simulink model "pv_partial_shading_control"  (R2021a)
settings: Solver=VariableStepAuto  StartTime=0.0  StopTime=2  RelTol=1e-3
libraries: pid_lib x5, spsSeriesRLCBranchLib x5, spsDiodeLib x4, spsabctodq0Lib x4, spsPVArrayLib x3, spsCurrentMeasurementLib x2, spsThreePhaseVIMeasurementLib x2, spsVoltageMeasurementLib x2, spsGroundLib x1, spsIGBTDiodeLib x1, spsPWMGenerator2LevelLib x1, spsPWMGeneratorDCDCLib x1
settings Model: Creator=30698  LastModifiedBy=30698
settings SolverCC: ZeroCrossAlgorithm=Adaptive
settings DebuggingCC: IgnoredZcDiagnostic=none  UnconnectedInputMsg=none  UnconnectedOutputMsg=none  UnconnectedLineMsg=none
settings ModelReferenceCC: EnableRefExpFcnMdlSchedulingChecks=off
settings RTWCC: Description=Generic Real-Time Target  DLArmComputeVersion=20.02.1

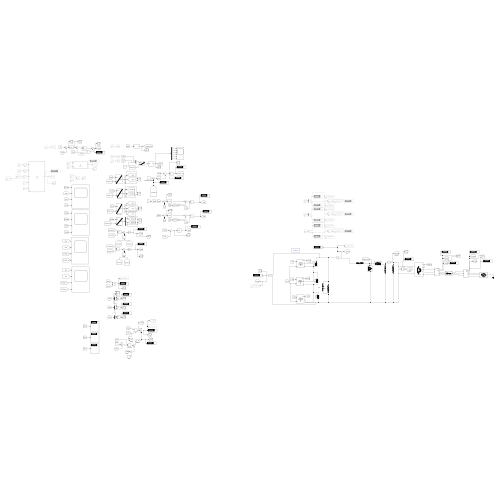
[thumbnail: Simulink's stored preview of the top-level diagram]
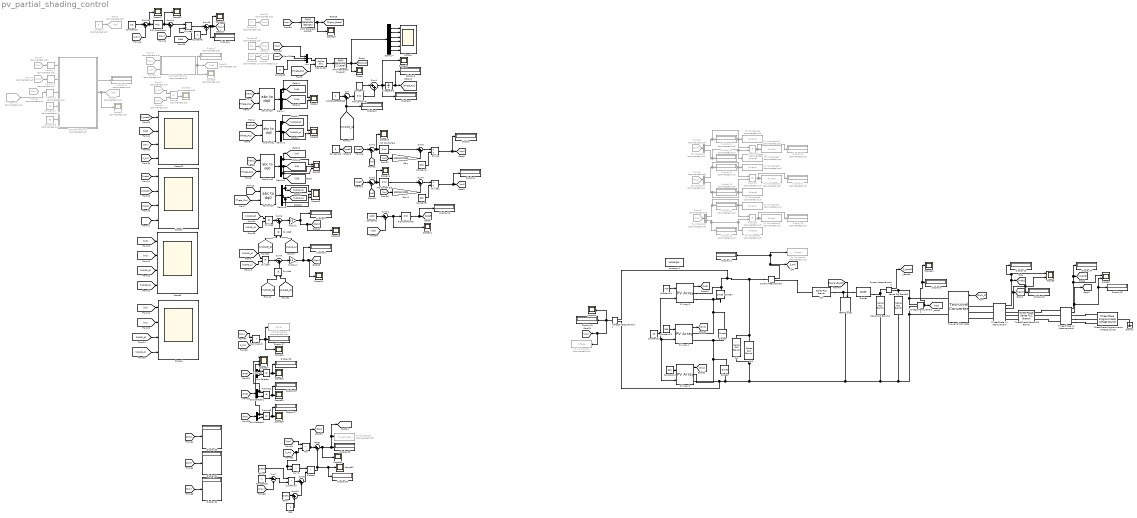
== system pv_partial_shading_control ==
  (1-d) : Sum  Inputs=|+-
  (1-d)Rdi,on : DotProduct  InputSameDT=on  OutDataTypeStr=Inherit: Inherit via internal rule
  Bus Selector : BusSelector  OutputSignals=V_PV,I_PV
  Bus Selector1 : BusSelector  OutputSignals=V_PV,I_PV
  Bus Selector2 : BusSelector  OutputSignals=V_PV,I_PV
  Bus Selector3 : BusSelector  Commented=on  OutputSignals=I_PV,V_PV
  Bus Selector4 : BusSelector  Commented=on  OutputSignals=I_PV,V_PV
  Bus Selector5 : BusSelector  Commented=on  OutputSignals=I_PV,V_PV
  Constant : Constant  Commented=on  Value=5
  Constant1 : Constant  Value=1200
  Constant10 : Constant  Value=0
  Constant11 : Constant  Value=700
  Constant12 : Constant  Value=350
  Constant13 : Constant  Value=25
  Constant14 : Constant  Value=600
  Constant15 : Constant  Value=25
  Constant16 : Constant  Commented=on  Value=55
  Constant17 : Constant  Commented=on  Value=30
  Constant18 : Constant
  Constant2 : Constant  Value=100*pi
  Constant3 : Constant  Value=0
  Constant4 : Constant  Value=600
  Constant5 : Constant  Value=600
  Constant6 : Constant
  Constant7 : Constant  Commented=on  Value=0.7
  Constant8 : Constant  Commented=on  Value=0.6
  Constant9 : Constant  Commented=on  Value=0.4
  Current Measurement : spsCurrentMeasurementLib/Current Measurement  PhasorSimulation=off  OutputType=Complex  PSBequivalent=0
  Current Measurement1 : spsCurrentMeasurementLib/Current Measurement  PhasorSimulation=off  OutputType=Complex  PSBequivalent=0
  Demux{,1..3} (4 alike) : Demux  Outputs=3
  Demux4 : Demux  Outputs=6
  Diode{1..4} (4 alike) : spsDiodeLib/Diode  Ron=0.001  Lon=0  Vf=0.8  IC=0  UseSnubber=0  Rs=500  Cs=250e-9  Measurements=on
  Display{,1..6,8..17,27..33,35} (25 alike) : Display
  Display{7,18..26,34} (11 alike) : Display  Commented=on
  Divide : Product  Inputs=*/
  Divide1 : Product  Inputs=*/
  Divide2 : Product  Inputs=*/
  Divide{3..6} (4 alike) : Product  Inputs=**
  Dot Product : DotProduct  InputSameDT=on  OutDataTypeStr=Inherit: Inherit via internal rule
  From36 : From  Commented=on  GotoTag=I_PV
  From37 : From  Commented=on  GotoTag=Vpv
  From38 : From  Commented=on  GotoTag=PV3
  From42 : From  Commented=on  GotoTag=PV2
  From43 : From  Commented=on  GotoTag=PV1
  From44 : From  Commented=on  GotoTag=I_PV
  From47 : From  Commented=on  GotoTag=I_PV
  From49 : From  Commented=on  GotoTag=V_PV
  From67 : From  Commented=on  GotoTag=Vpv
  From69 : From  Commented=on  GotoTag=Ppv
  From70 : From  Commented=on  GotoTag=Ppv_Losses
  Gain : Gain  Gain=100*pi*0.001
  Gain1 : Gain  Gain=100*pi*0.001
  Goto24 : Goto  Commented=on  GotoTag=Iref
  Goto26 : Goto  Commented=on  GotoTag=mpv
  Goto27 : Goto  Commented=on  GotoTag=md
  Goto28 : Goto  Commented=on  GotoTag=mq
  Goto32 : Goto  Commented=on  GotoTag=Iref
  Goto5 : Goto  Commented=on  GotoTag=Iref
  Ground : spsGroundLib/Ground  LConnTagsString=a
  IGBT/Diode1 : spsIGBTDiodeLib/IGBT//Diode  Ron=1e-3  Rs=1e5  Cs=inf  Measurements=off
  Integrator2 : Integrator
  Ipv^2 : DotProduct  InputSameDT=on  OutDataTypeStr=Inherit: Inherit via internal rule
  MATLAB Function1 : MATLAB Function  Commented=on  TreatAsAtomicUnit=on
  MATLAB Function4 : MATLAB Function  Commented=on  TreatAsAtomicUnit=on
      settings: MinAlgLoopOccurrences=on
  Memory1 : Memory  Commented=on  InheritSampleTime=on
  Memory2 : Memory  Commented=on  InheritSampleTime=on
  Memory3 : Memory  Commented=on  InheritSampleTime=on
  Multiply : Gain  Gain=1.5
  Multiply1 : Gain  Gain=1.5
  Mux : Mux  Inputs=3
  PID Controller : pid_lib/PID Controller  Controller=PI  Form=Parallel  TimeDomain=Continuous-time  UseExternalTs=off  SampleTime=-1  IntegratorMethod=Forward Euler  FilterMethod=Forward Euler  ControllerParametersSource=internal  P=18  I=320  D=0  N=100  UseFilter=on  TunerSelectOption=Transfer Function Based (PID Tuner App)  InitialConditionSource=internal  InitialConditionForIntegrator=0  InitialConditionForFilter=0  DifferentiatorICPrevScaledInput=0  ExternalReset=none  TrackingMode=off  Kt=1  LimitOutput=off  SatLimitsSource=internal  UpperSaturationLimit=inf  LowerSaturationLimit=-inf  LinearizeAsGain=on  AntiWindupMode=none  Kb=1  POutMin=[]  POutMax=[]  IOutMin=[]  IOutMax=[]  DOutMin=[]  DOutMax=[]  NOutMin=[]  NOutMax=[]  SumOutMin=[]  SumOutMax=[]  SaturationOutMin=[]  SaturationOutMax=[]  PParamMin=[]  PParamMax=[]  IParamMin=[]  IParamMax=[]  DParamMin=[]  DParamMax=[]  NParamMin=[]  NParamMax=[]  KbParamMin=[]  KbParamMax=[]  KtParamMin=[]  KtParamMax=[]  KbOutMin=[]  KbOutMax=[]  KtOutMin=[]  KtOutMax=[]  IntegratorOutMin=[]  IntegratorOutMax=[]  FilterOutMin=[]  FilterOutMax=[]  SumI1OutMin=[]  SumI1OutMax=[]  SumI2OutMin=[]  SumI2OutMax=[]  SumI3OutMin=[]  SumI3OutMax=[]  SumI4OutMin=[]  SumI4OutMax=[]  SumDOutMin=[]  SumDOutMax=[]  DifferentiatorOutMin=[]  DifferentiatorOutMax=[]  FilterDiffOutCoefMin=[]  FilterDiffOutCoefMax=[]  ReciprocalOutMin=[]  ReciprocalOutMax=[]  SumDenOutMin=[]  SumDenOutMax=[]  SumNumOutMin=[]  SumNumOutMax=[]  DivideOutMin=[]  DivideOutMax=[]  UdiffTsProdOutMin=[]  UdiffTsProdOutMax=[]  NTsProdOutMin=[]  NTsProdOutMax=[]  UintegralTsProdOutMin=[]  UintegralTsProdOutMax=[]  UngainTsProdOutMin=[]  UngainTsProdOutMax=[]  IntegratorContinuousStateAttributes=''  IntegratorStateMustResolveToSignalObject=off  IntegratorRTWStateStorageClass=Auto  FilterContinuousStateAttributes=''  FilterStateMustResolveToSignalObject=off  FilterRTWStateStorageClass=Auto  ParallelPVariant=InternalParameters  IdealPVariant=Disabled  IVariant=InternalParameters  DVariant=Disabled  IntegratorVariant=Continuous  SatVariant=Disabled  AWVariant=Passthrough  PCopyVariant=Disabled  TRVariant=Disabled  FdbkBlocksVariant=Forward  IdealPFdbkVariant=Disabled  SatFdbkVariant=Disabled  DerivativeFilterVariant=Disabled  NVariant=Disabled  NCopyVariant=Disabled_SignalSpec  FilterICVariant=Disabled  IntegratorICVariant=InternalICs  ExternalResetVariant=Disabled  TRSumVariant=Passthrough  SumFdbkVariant=Disabled  SumVariant=Sum_PI  TsampFilterVariant=InternalTs  TsampNgainVariant=Passthrough  TsampIntegralVariant=Disabled_SignalSpec  ExternalSaturationOutDataTypeStr=Inherit: Same as second input
  PID Controller1 : pid_lib/PID Controller  Controller=PI  Form=Parallel  TimeDomain=Continuous-time  UseExternalTs=off  SampleTime=-1  IntegratorMethod=Forward Euler  FilterMethod=Forward Euler  ControllerParametersSource=internal  P=5  I=50  D=0  N=100  UseFilter=on  TunerSelectOption=Transfer Function Based (PID Tuner App)  InitialConditionSource=internal  InitialConditionForIntegrator=0  InitialConditionForFilter=0  DifferentiatorICPrevScaledInput=0  ExternalReset=none  TrackingMode=off  Kt=1  LimitOutput=off  SatLimitsSource=internal  UpperSaturationLimit=inf  LowerSaturationLimit=-inf  LinearizeAsGain=on  AntiWindupMode=none  Kb=1  POutMin=[]  POutMax=[]  IOutMin=[]  IOutMax=[]  DOutMin=[]  DOutMax=[]  NOutMin=[]  NOutMax=[]  SumOutMin=[]  SumOutMax=[]  SaturationOutMin=[]  SaturationOutMax=[]  PParamMin=[]  PParamMax=[]  IParamMin=[]  IParamMax=[]  DParamMin=[]  DParamMax=[]  NParamMin=[]  NParamMax=[]  KbParamMin=[]  KbParamMax=[]  KtParamMin=[]  KtParamMax=[]  KbOutMin=[]  KbOutMax=[]  KtOutMin=[]  KtOutMax=[]  IntegratorOutMin=[]  IntegratorOutMax=[]  FilterOutMin=[]  FilterOutMax=[]  SumI1OutMin=[]  SumI1OutMax=[]  SumI2OutMin=[]  SumI2OutMax=[]  SumI3OutMin=[]  SumI3OutMax=[]  SumI4OutMin=[]  SumI4OutMax=[]  SumDOutMin=[]  SumDOutMax=[]  DifferentiatorOutMin=[]  DifferentiatorOutMax=[]  FilterDiffOutCoefMin=[]  FilterDiffOutCoefMax=[]  ReciprocalOutMin=[]  ReciprocalOutMax=[]  SumDenOutMin=[]  SumDenOutMax=[]  SumNumOutMin=[]  SumNumOutMax=[]  DivideOutMin=[]  DivideOutMax=[]  UdiffTsProdOutMin=[]  UdiffTsProdOutMax=[]  NTsProdOutMin=[]  NTsProdOutMax=[]  UintegralTsProdOutMin=[]  UintegralTsProdOutMax=[]  UngainTsProdOutMin=[]  UngainTsProdOutMax=[]  IntegratorContinuousStateAttributes=''  IntegratorStateMustResolveToSignalObject=off  IntegratorRTWStateStorageClass=Auto  FilterContinuousStateAttributes=''  FilterStateMustResolveToSignalObject=off  FilterRTWStateStorageClass=Auto  ParallelPVariant=InternalParameters  IdealPVariant=Disabled  IVariant=InternalParameters  DVariant=Disabled  IntegratorVariant=Continuous  SatVariant=Disabled  AWVariant=Passthrough  PCopyVariant=Disabled  TRVariant=Disabled  FdbkBlocksVariant=Forward  IdealPFdbkVariant=Disabled  SatFdbkVariant=Disabled  DerivativeFilterVariant=Disabled  NVariant=Disabled  NCopyVariant=Disabled_SignalSpec  FilterICVariant=Disabled  IntegratorICVariant=InternalICs  ExternalResetVariant=Disabled  TRSumVariant=Passthrough  SumFdbkVariant=Disabled  SumVariant=Sum_PI  TsampFilterVariant=InternalTs  TsampNgainVariant=Passthrough  TsampIntegralVariant=Disabled_SignalSpec  ExternalSaturationOutDataTypeStr=Inherit: Same as second input
  PID Controller2 : pid_lib/PID Controller  Controller=PI  Form=Parallel  TimeDomain=Continuous-time  UseExternalTs=off  SampleTime=-1  IntegratorMethod=Forward Euler  FilterMethod=Forward Euler  ControllerParametersSource=internal  P=5  I=50  D=0  N=100  UseFilter=on  TunerSelectOption=Transfer Function Based (PID Tuner App)  InitialConditionSource=internal  InitialConditionForIntegrator=0  InitialConditionForFilter=0  DifferentiatorICPrevScaledInput=0  ExternalReset=none  TrackingMode=off  Kt=1  LimitOutput=off  SatLimitsSource=internal  UpperSaturationLimit=inf  LowerSaturationLimit=-inf  LinearizeAsGain=on  AntiWindupMode=none  Kb=1  POutMin=[]  POutMax=[]  IOutMin=[]  IOutMax=[]  DOutMin=[]  DOutMax=[]  NOutMin=[]  NOutMax=[]  SumOutMin=[]  SumOutMax=[]  SaturationOutMin=[]  SaturationOutMax=[]  PParamMin=[]  PParamMax=[]  IParamMin=[]  IParamMax=[]  DParamMin=[]  DParamMax=[]  NParamMin=[]  NParamMax=[]  KbParamMin=[]  KbParamMax=[]  KtParamMin=[]  KtParamMax=[]  KbOutMin=[]  KbOutMax=[]  KtOutMin=[]  KtOutMax=[]  IntegratorOutMin=[]  IntegratorOutMax=[]  FilterOutMin=[]  FilterOutMax=[]  SumI1OutMin=[]  SumI1OutMax=[]  SumI2OutMin=[]  SumI2OutMax=[]  SumI3OutMin=[]  SumI3OutMax=[]  SumI4OutMin=[]  SumI4OutMax=[]  SumDOutMin=[]  SumDOutMax=[]  DifferentiatorOutMin=[]  DifferentiatorOutMax=[]  FilterDiffOutCoefMin=[]  FilterDiffOutCoefMax=[]  ReciprocalOutMin=[]  ReciprocalOutMax=[]  SumDenOutMin=[]  SumDenOutMax=[]  SumNumOutMin=[]  SumNumOutMax=[]  DivideOutMin=[]  DivideOutMax=[]  UdiffTsProdOutMin=[]  UdiffTsProdOutMax=[]  NTsProdOutMin=[]  NTsProdOutMax=[]  UintegralTsProdOutMin=[]  UintegralTsProdOutMax=[]  UngainTsProdOutMin=[]  UngainTsProdOutMax=[]  IntegratorContinuousStateAttributes=''  IntegratorStateMustResolveToSignalObject=off  IntegratorRTWStateStorageClass=Auto  FilterContinuousStateAttributes=''  FilterStateMustResolveToSignalObject=off  FilterRTWStateStorageClass=Auto  ParallelPVariant=InternalParameters  IdealPVariant=Disabled  IVariant=InternalParameters  DVariant=Disabled  IntegratorVariant=Continuous  SatVariant=Disabled  AWVariant=Passthrough  PCopyVariant=Disabled  TRVariant=Disabled  FdbkBlocksVariant=Forward  IdealPFdbkVariant=Disabled  SatFdbkVariant=Disabled  DerivativeFilterVariant=Disabled  NVariant=Disabled  NCopyVariant=Disabled_SignalSpec  FilterICVariant=Disabled  IntegratorICVariant=InternalICs  ExternalResetVariant=Disabled  TRSumVariant=Passthrough  SumFdbkVariant=Disabled  SumVariant=Sum_PI  TsampFilterVariant=InternalTs  TsampNgainVariant=Passthrough  TsampIntegralVariant=Disabled_SignalSpec  ExternalSaturationOutDataTypeStr=Inherit: Same as second input
  PID Controller3 : pid_lib/PID Controller  Controller=PI  Form=Parallel  TimeDomain=Continuous-time  UseExternalTs=off  SampleTime=-1  IntegratorMethod=Forward Euler  FilterMethod=Forward Euler  ControllerParametersSource=internal  P=-10  I=-200  D=0  N=100  UseFilter=on  TunerSelectOption=Transfer Function Based (PID Tuner App)  InitialConditionSource=internal  InitialConditionForIntegrator=0  InitialConditionForFilter=0  DifferentiatorICPrevScaledInput=0  ExternalReset=none  TrackingMode=off  Kt=1  LimitOutput=off  SatLimitsSource=internal  UpperSaturationLimit=inf  LowerSaturationLimit=-inf  LinearizeAsGain=on  AntiWindupMode=none  Kb=1  POutMin=[]  POutMax=[]  IOutMin=[]  IOutMax=[]  DOutMin=[]  DOutMax=[]  NOutMin=[]  NOutMax=[]  SumOutMin=[]  SumOutMax=[]  SaturationOutMin=[]  SaturationOutMax=[]  PParamMin=[]  PParamMax=[]  IParamMin=[]  IParamMax=[]  DParamMin=[]  DParamMax=[]  NParamMin=[]  NParamMax=[]  KbParamMin=[]  KbParamMax=[]  KtParamMin=[]  KtParamMax=[]  KbOutMin=[]  KbOutMax=[]  KtOutMin=[]  KtOutMax=[]  IntegratorOutMin=[]  IntegratorOutMax=[]  FilterOutMin=[]  FilterOutMax=[]  SumI1OutMin=[]  SumI1OutMax=[]  SumI2OutMin=[]  SumI2OutMax=[]  SumI3OutMin=[]  SumI3OutMax=[]  SumI4OutMin=[]  SumI4OutMax=[]  SumDOutMin=[]  SumDOutMax=[]  DifferentiatorOutMin=[]  DifferentiatorOutMax=[]  FilterDiffOutCoefMin=[]  FilterDiffOutCoefMax=[]  ReciprocalOutMin=[]  ReciprocalOutMax=[]  SumDenOutMin=[]  SumDenOutMax=[]  SumNumOutMin=[]  SumNumOutMax=[]  DivideOutMin=[]  DivideOutMax=[]  UdiffTsProdOutMin=[]  UdiffTsProdOutMax=[]  NTsProdOutMin=[]  NTsProdOutMax=[]  UintegralTsProdOutMin=[]  UintegralTsProdOutMax=[]  UngainTsProdOutMin=[]  UngainTsProdOutMax=[]  IntegratorContinuousStateAttributes=''  IntegratorStateMustResolveToSignalObject=off  IntegratorRTWStateStorageClass=Auto  FilterContinuousStateAttributes=''  FilterStateMustResolveToSignalObject=off  FilterRTWStateStorageClass=Auto  ParallelPVariant=InternalParameters  IdealPVariant=Disabled  IVariant=InternalParameters  DVariant=Disabled  IntegratorVariant=Continuous  SatVariant=Disabled  AWVariant=Passthrough  PCopyVariant=Disabled  TRVariant=Disabled  FdbkBlocksVariant=Forward  IdealPFdbkVariant=Disabled  SatFdbkVariant=Disabled  DerivativeFilterVariant=Disabled  NVariant=Disabled  NCopyVariant=Disabled_SignalSpec  FilterICVariant=Disabled  IntegratorICVariant=InternalICs  ExternalResetVariant=Disabled  TRSumVariant=Passthrough  SumFdbkVariant=Disabled  SumVariant=Sum_PI  TsampFilterVariant=InternalTs  TsampNgainVariant=Passthrough  TsampIntegralVariant=Disabled_SignalSpec  ExternalSaturationOutDataTypeStr=Inherit: Same as second input
  PID Controller4 : pid_lib/PID Controller  Controller=PI  Form=Parallel  TimeDomain=Continuous-time  UseExternalTs=off  SampleTime=-1  IntegratorMethod=Forward Euler  FilterMethod=Forward Euler  ControllerParametersSource=internal  P=10  I=1500  D=0  N=100  UseFilter=on  TunerSelectOption=Frequency Response Based  InitialConditionSource=internal  InitialConditionForIntegrator=0  InitialConditionForFilter=0  DifferentiatorICPrevScaledInput=0  ExternalReset=none  TrackingMode=off  Kt=1  LimitOutput=off  SatLimitsSource=internal  UpperSaturationLimit=inf  LowerSaturationLimit=-inf  LinearizeAsGain=on  AntiWindupMode=none  Kb=1  POutMin=[]  POutMax=[]  IOutMin=[]  IOutMax=[]  DOutMin=[]  DOutMax=[]  NOutMin=[]  NOutMax=[]  SumOutMin=[]  SumOutMax=[]  SaturationOutMin=[]  SaturationOutMax=[]  PParamMin=[]  PParamMax=[]  IParamMin=[]  IParamMax=[]  DParamMin=[]  DParamMax=[]  NParamMin=[]  NParamMax=[]  KbParamMin=[]  KbParamMax=[]  KtParamMin=[]  KtParamMax=[]  KbOutMin=[]  KbOutMax=[]  KtOutMin=[]  KtOutMax=[]  IntegratorOutMin=[]  IntegratorOutMax=[]  FilterOutMin=[]  FilterOutMax=[]  SumI1OutMin=[]  SumI1OutMax=[]  SumI2OutMin=[]  SumI2OutMax=[]  SumI3OutMin=[]  SumI3OutMax=[]  SumI4OutMin=[]  SumI4OutMax=[]  SumDOutMin=[]  SumDOutMax=[]  DifferentiatorOutMin=[]  DifferentiatorOutMax=[]  FilterDiffOutCoefMin=[]  FilterDiffOutCoefMax=[]  ReciprocalOutMin=[]  ReciprocalOutMax=[]  SumDenOutMin=[]  SumDenOutMax=[]  SumNumOutMin=[]  SumNumOutMax=[]  DivideOutMin=[]  DivideOutMax=[]  UdiffTsProdOutMin=[]  UdiffTsProdOutMax=[]  NTsProdOutMin=[]  NTsProdOutMax=[]  UintegralTsProdOutMin=[]  UintegralTsProdOutMax=[]  UngainTsProdOutMin=[]  UngainTsProdOutMax=[]  IntegratorContinuousStateAttributes=''  IntegratorStateMustResolveToSignalObject=off  IntegratorRTWStateStorageClass=Auto  FilterContinuousStateAttributes=''  FilterStateMustResolveToSignalObject=off  FilterRTWStateStorageClass=Auto  ParallelPVariant=InternalParameters  IdealPVariant=Disabled  IVariant=InternalParameters  DVariant=Disabled  IntegratorVariant=Continuous  SatVariant=Disabled  AWVariant=Passthrough  PCopyVariant=Disabled  TRVariant=Disabled  FdbkBlocksVariant=Forward  IdealPFdbkVariant=Disabled  SatFdbkVariant=Disabled  DerivativeFilterVariant=Disabled  NVariant=Disabled  NCopyVariant=Disabled_SignalSpec  FilterICVariant=Disabled  IntegratorICVariant=InternalICs  ExternalResetVariant=Disabled  TRSumVariant=Passthrough  SumFdbkVariant=Disabled  SumVariant=Sum_PI  TsampFilterVariant=InternalTs  TsampNgainVariant=Passthrough  TsampIntegralVariant=Disabled_SignalSpec  ExternalSaturationOutDataTypeStr=Inherit: Same as second input
  PV Array1 : spsPVArrayLib/PV Array  Npar=10  Nser=6  PlotType=array @ 1000 W/m2 & specified temperatures  S_vec="[ 1000  500  100 ]"  Temp_C_vec="[ 45 25  ]"  ModuleName=User-defined  PlotWhenSelected=off  Pm=213.15  Ncell=60  Voc=36.3  Isc=7.84  Vm=29  Im=7.35  beta_Voc_pc=-0.36099  alpha_Isc_pc=0.102  beta_Voc=-0.13104  alpha_Isc=0.0079968  IL=7.8654  I0=2.9273e-10  nI=0.98119  Rsh=313.0553  Rs=0.39381  RobustModel=off  RobustCellTemperature=25  BAL=on  Tc=1e-6  Tfilter=5e-5
  PV Array2 : spsPVArrayLib/PV Array  Npar=10  Nser=7  PlotType=array @ 1000 W/m2 & specified temperatures  S_vec="[ 1000  500  100 ]"  Temp_C_vec="[ 45 25  ]"  ModuleName=User-defined  PlotWhenSelected=off  Pm=213.15  Ncell=60  Voc=36.3  Isc=7.84  Vm=29  Im=7.35  beta_Voc_pc=-0.36099  alpha_Isc_pc=0.102  beta_Voc=-0.13104  alpha_Isc=0.0079968  IL=7.8654  I0=2.9273e-10  nI=0.98119  Rsh=313.0553  Rs=0.39381  RobustModel=off  RobustCellTemperature=25  BAL=on  Tc=1e-6  Tfilter=5e-5
  PV Array3 : spsPVArrayLib/PV Array  Npar=10  Nser=4  PlotType=array @ 1000 W/m2 & specified temperatures  S_vec="[ 1000  500  100 ]"  Temp_C_vec="[ 45 25  ]"  ModuleName=User-defined  PlotWhenSelected=off  Pm=213.15  Ncell=60  Voc=36.3  Isc=7.84  Vm=29  Im=7.35  beta_Voc_pc=-0.36099  alpha_Isc_pc=0.102  beta_Voc=-0.13104  alpha_Isc=0.0079968  IL=7.8654  I0=2.9273e-10  nI=0.98119  Rsh=313.0553  Rs=0.39381  RobustModel=off  RobustCellTemperature=25  BAL=on  Tc=1e-6  Tfilter=5e-5
  PWM Generator (2-Level) : spsPWMGenerator2LevelLib/PWM Generator (2-Level)  ModulatorType=Three-phase bridge (6 pulses)  ModulatorMode=Unsynchronized  Fc=61*50  Pc=90  nF=27  MinMax="[ -1  1 ]"  SamplingTechnique=Natural  ModulatingSignals=off  m=0.8  Freq=60  Phase=0  Ts=0  ShowCarrierOutport=off
  PWM Generator (DC-DC) : spsPWMGeneratorDCDCLib/PWM Generator (DC-DC)  Fsw=40000  Ts=0
  Plosses : DotProduct  InputSameDT=on  OutDataTypeStr=Inherit: Inherit via internal rule
  Ppv : DotProduct  InputSameDT=on  OutDataTypeStr=Inherit: Inherit via internal rule
  Product{,3..5} (4 alike) : Product  Commented=on
  Product1 : Product
  Product2 : Product
  Product6 : Product
  Ptotal : Sum  Inputs=|+-
  RL1 : spsSeriesRLCBranchLib/Series RLC Branch  LConnTagsString=__new0  RConnTagsString=__new0  BranchType=RL  Resistance=0.1  Inductance=2e-3  SetiL0=off  InitialCurrent=0  Capacitance=1e-6  Setx0=off  InitialVoltage=0  Measurements=None
  RL2 : spsSeriesRLCBranchLib/Series RLC Branch  LConnTagsString=__new0  RConnTagsString=__new0  BranchType=C  Resistance=0.1  Inductance=1.5e-3  SetiL0=off  InitialCurrent=0  Capacitance=1e-9  Setx0=on  InitialVoltage=50  Measurements=None
  RL3 : spsSeriesRLCBranchLib/Series RLC Branch  LConnTagsString=__new0  RConnTagsString=__new0  BranchType=R  Resistance=10000  Inductance=1.5e-3  SetiL0=off  InitialCurrent=0  Capacitance=1e-9  Setx0=on  InitialVoltage=50  Measurements=None
  Rdi,on : Constant  Value=0.001
  Req : Constant
  Rtr,on : Constant  Value=0.001
  Scope{,11,13..17,19..22,24..26,28..30,32..33} (19 alike) : Scope
  Scope1 : Scope  NumInputPorts=6
  Scope10 : Scope  NumInputPorts=3
  Scope{2..4,12} (4 alike) : Scope  NumInputPorts=4
  Scope18 : Scope  Commented=on
  Scope23 : Scope  Commented=on
  Scope27 : Scope  NumInputPorts=3
  Scope31 : Scope  Commented=on
  Scope{5..8} (4 alike) : Scope  NumInputPorts=2
  Scope9 : Scope  NumInputPorts=3
  Series RLC Branch2 : spsSeriesRLCBranchLib/Series RLC Branch  LConnTagsString=__new0  RConnTagsString=__new0  BranchType=C  Resistance=1  Inductance=1e-3  SetiL0=off  InitialCurrent=0  Capacitance=1e-3  Setx0=on  InitialVoltage=1200  Measurements=None
  Series RLC Branch3 : spsSeriesRLCBranchLib/Series RLC Branch  LConnTagsString=__new0  RConnTagsString=__new0  BranchType=R  Resistance=100  Inductance=1e-3  SetiL0=off  InitialCurrent=0  Capacitance=1e-6  Setx0=off  InitialVoltage=0  Measurements=None
  Sum{,1,5..6,8,10,15} (7 alike) : Sum  Inputs=|++
  Sum{2..4,12..14} (6 alike) : Sum  Inputs=|+-
  Sum9 : Sum  Inputs=|-+
  Three-Phase Programmable Voltage Source : spsThreePhaseProgrammableVoltageSourceLib/Three-Phase Programmable Voltage Source  PositiveSequence=[400 30 50]  VariationEntity=None  VariationType=Table of time-amplitude pairs  VariationTypeAlt=Step  VariationStep=0.5  VariationRate=10  VariationMagnitude=0.3  VariationFrequency=2  VariationTiming=[1 2]  VariationPhaseA=off  Amplitudes=[1 0.8 1.2 1.0]  TimeValues=[0 0.1 0.15 0.2]  HarmonicGeneration=off  HarmonicA=[3 0.2 -25 0]  HarmonicB=[2 0.15 35 2]  Timing="[0.05  3]"  BusType=swing  Pref=0  Qref=0  Qmin=-inf  Qmax=inf
  Three-Phase Series RLC Branch : spsThreePhaseSeriesRLCBranchLib/Three-Phase Series RLC Branch  LConnTagsString=A|B|C  RConnTagsString=A|B|C  BranchType=RL  Resistance=0.01  Inductance=1e-3  Capacitance=1e-6  Measurements=None
  Three-Phase V-I Measurement : spsThreePhaseVIMeasurementLib/Three-Phase V-I Measurement  VoltageMeasurement=phase-to-ground  SetLabelV=off  LabelV=Vabc  Vpu=off  VpuLL=off  CurrentMeasurement=yes  SetLabelI=off  LabelI=Iabc  Ipu=off  Pbase=100e6  Vbase=500e3  OutputType=Complex  PhasorSimulation=off  PSBequivalent=0
  Three-Phase V-I Measurement1 : spsThreePhaseVIMeasurementLib/Three-Phase V-I Measurement  VoltageMeasurement=phase-to-ground  SetLabelV=off  LabelV=Vabc  Vpu=off  VpuLL=off  CurrentMeasurement=yes  SetLabelI=off  LabelI=Iabc  Ipu=off  Pbase=100e6  Vbase=500e3  OutputType=Complex  PhasorSimulation=off  PSBequivalent=0
  To Workspace : ToWorkspace  Commented=on  VariableName=Current  SampleTime=-1
      settings: Save2DSignal=2-D array (concatenate along first dimension)
  To Workspace1 : ToWorkspace  Commented=on  VariableName=PowerLosses  SampleTime=-1
      settings: Save2DSignal=2-D array (concatenate along first dimension)
  To Workspace10 : ToWorkspace  Commented=on  VariableName=Power1  SampleTime=-1
      settings: Save2DSignal=2-D array (concatenate along first dimension)
  To Workspace11 : ToWorkspace  Commented=on  VariableName=Power2  SampleTime=-1
      settings: Save2DSignal=2-D array (concatenate along first dimension)
  To Workspace12 : ToWorkspace  Commented=on  VariableName=Power3  SampleTime=-1
      settings: Save2DSignal=2-D array (concatenate along first dimension)
  To Workspace2 : ToWorkspace  Commented=on  VariableName=Power  SampleTime=-1
      settings: Save2DSignal=2-D array (concatenate along first dimension)
  To Workspace3 : ToWorkspace  Commented=on  VariableName=Voltage  SampleTime=-1
      settings: Save2DSignal=2-D array (concatenate along first dimension)
  To Workspace4 : ToWorkspace  Commented=on  VariableName=Current1  SampleTime=-1
      settings: Save2DSignal=2-D array (concatenate along first dimension)
  To Workspace5 : ToWorkspace  Commented=on  VariableName=Current2  SampleTime=-1
      settings: Save2DSignal=2-D array (concatenate along first dimension)
  To Workspace6 : ToWorkspace  Commented=on  VariableName=Current3  SampleTime=-1
      settings: Save2DSignal=2-D array (concatenate along first dimension)
  To Workspace7 : ToWorkspace  Commented=on  VariableName=Voltage1  SampleTime=-1
      settings: Save2DSignal=2-D array (concatenate along first dimension)
  To Workspace8 : ToWorkspace  Commented=on  VariableName=Voltage2  SampleTime=-1
      settings: Save2DSignal=2-D array (concatenate along first dimension)
  To Workspace9 : ToWorkspace  Commented=on  VariableName=Voltage3  SampleTime=-1
      settings: Save2DSignal=2-D array (concatenate along first dimension)
  Two-Level Converter : spsTwoLevelConverterLib/Two-Level Converter  ModelType=Switching devices  Ron=1e-3  Rs=1e6  Cs=inf  Vforward=[0,0]  Ron_Diode=1e-3  Rs_Diode=1e6  Cs_Diode=inf  Vf_Diode=1e-3  Rs_CurrentSource=inf  Ron_ACsource=1e-3
  VLOAD-REFERENCE : Constant  Value=0
  Voltage Measurement1 : spsVoltageMeasurementLib/Voltage Measurement  PhasorSimulation=off  OutputType=Complex  PSBequivalent=0
  Voltage Measurement2 : spsVoltageMeasurementLib/Voltage Measurement  PhasorSimulation=off  OutputType=Complex  PSBequivalent=0
  abc to dq{0..3} (4 alike) : spsabctodq0Lib/abc to dq0  Alignment=90 degrees behind phase A axis
  dq0 to abc : spsdq0toabcLib/dq0 to abc  Alignment=90 degrees behind phase A axis
  powergui1 : spspowerguiLib/powergui  Priority=1  SimulationMode=Continuous  SampleTime=1e-5  frequency=60  Iterations=50  frequencyindice=0  Pbase=100e6  ErrMax=1e-4  UnitsV=kV  UnitsW=MW  buscounter=0  FunctionMessages=off  echomessages=off  EnableUseOfTLC=off  CurrentSourceSwitches=off  DisableSnubberDevices=off  DisableRonSwitches=off  DisableVfSwitches=off  DisplayEquations=off  AutomaticDiscreteSolvers=off  SolverType=Tustin/Backward Euler (TBE)  Interpol=off  ExternalGateDelay=off  methode=off  Ts=100  x0status=blocks  SPID=on  SwTol=0  HookPort=off  NonlinearTolerance=1e-4  nMaxIteration=100  ContinueOnMaxIteration=off  RestoreLinks=warning  ResistiveCurrentMeasurement=off  Frange=[0:2:500]  Ylog=off  Xlog=on  ShowGrid=off  save=off  variable=ZData  structure=0  ZoomFFT=off  StartTime=0.0  cycles=1  DisplayStyle=1  fundamental=60  FreqAxis=off  MaxFrequency=1000  frequencyindicesteady=1  RmsSteady=1  display=off
  wires:
  [Theta_PLL] -> dq0 to abc/2
  Demux4/5 -> Scope1/5
  Divide5/1 -> Sum6/2
  [IIabc] -> abc to dq2/1
  Three-Phase V-I Measurement/1 -> Display12/1, Scope5/1, [VIabc]
  Demux3/3 -> Scope10/3
  [IIq] -> Sum2/2
  [IIabc] -> Scope2/3
  Sum9/1 -> Multiply1/1
  [PWM_1] -> Two-Level Converter/1
  Mux/1 -> dq0 to abc/1
  Gain/1 -> Sum5/2
  Constant5/1 -> Divide1/2
  Demux3/2 -> [ILOAD_q], Scope10/2
  Demux2/3 -> Scope9/3, [II0]
  Sum2/1 -> Scope15/1, PID Controller1/1
  [Idref] -> Sum3/1
  [ILOAD] -> Scope2/4
  [VIq] -> Scope3/2
  Gain1/1 -> Sum4/2
  [Theta_PLL] -> abc to dq2/2
  [ILOAD] -> abc to dq3/1
  Constant4/1 -> Divide/2
  Sum3/1 -> Scope16/1, PID Controller2/1
  PID Controller1/1 -> Sum5/1
  Multiply1/1 -> Display5/1, Scope14/1, [Qgrid]
  Demux1/2 -> Scope8/2, [VLOAD_q]
  Sum5/1 -> Divide/1
  [Iqref] -> Sum2/1
  [IId] -> Gain/1
  [IId] -> Sum3/2
  [VLOAD_d] -> Scope3/3
  [VLOAD] -> Scope2/2
  dq0 to abc/1 -> PWM Generator (2-Level)/1
  [ILOAD_q] -> Scope4/4
  [IIq] -> Scope4/2
  [Theta_PLL] -> abc to dq3/2
  Sum1/1 -> Display8/1, Integrator2/1, Scope20/1
  [VLOAD_q] -> Scope3/4
  [IId] -> Scope4/1
  Demux/2 -> [VIq], Scope7/2
  [VId] -> Scope3/1
  Sum4/1 -> Divide1/1
  Sum6/1 -> Multiply/1
  Integrator2/1 -> Display2/1, [Theta_PLL]
  Demux2/1 -> Scope9/1, [IId]
  Demux4/2 -> Scope1/2
  Demux3/1 -> [ILOAD_d], Scope10/1
  Sum/1 -> PID Controller/1
  Demux4/1 -> Scope1/1
  [VLOAD_q] -> Sum/2, Display3/1
  VLOAD-REFERENCE/1 -> Sum/1
  Demux4/4 -> Scope1/4
  Divide3/1 -> Sum9/1
  Demux4/3 -> Scope1/3
  Demux4/6 -> Scope1/6
  abc to dq3/1 -> Demux3/1
  Three-Phase V-I Measurement/2 -> Scope5/2, Display13/1, [IIabc]
  Demux/1 -> [VId], Scope7/1
  abc to dq1/1 -> Demux1/1
  [Theta_PLL] -> abc to dq0/2
  Demux2/2 -> Scope9/2, [IIq]
  Multiply/1 -> Display4/1, Scope13/1, [Pgrid]
  PID Controller2/1 -> Sum4/1
  Demux1/1 -> Scope8/1, [VLOAD_d]
  Constant2/1 -> Sum1/1
  abc to dq2/1 -> Demux2/1
  Sum12/1 -> Scope11/1, PID Controller3/1
  [md] -> Mux/1
  [IIq] -> Gain1/1
  Constant3/1 -> Mux/3
  [Vdc] -> Sum12/2
  PID Controller3/1 -> Display16/1, [Idref]
  Three-Phase V-I Measurement1/2 -> Display15/1, Scope6/2, [ILOAD]
  Constant1/1 -> Sum12/1
  PWM Generator (2-Level)/1 -> [PWM_1], Scope/1, Demux4/1
  [Theta_PLL] -> abc to dq1/2
  [VLOAD] -> abc to dq1/1
  [ILOAD_d] -> Scope4/3
  Three-Phase V-I Measurement1/1 -> Scope6/1, Display14/1, [VLOAD]
  [VLOAD_d] -> Divide6/1
  [VIabc] -> abc to dq0/1
  abc to dq0/1 -> Demux/1
  [mq] -> Mux/2
  [VLOAD_d] -> Divide3/1
  [VIabc] -> Scope2/1
  Constant15/1 -> Sum13/1
  [Vpv] -> Scope12/3
  [Signal_Boost] -> IGBT/Diode1/1
  Divide2/1 -> Sum15/1
  PWM Generator (DC-DC)/1 -> Scope19/1, [Signal_Boost]
  Voltage Measurement2/1 -> Scope21/1, Display9/1, [Vdc]
  [mpv] -> PWM Generator (DC-DC)/1
  From47/1 -> Product/1
  Sum15/1 -> Scope22/1, [mpv], Display6/1
  [Vdc] -> Scope12/2
  From49/1 -> Product/2
  Product/1 -> Scope18/1
  [I_PV] -> Scope12/4
  Sum13/1 -> Scope17/1, PID Controller4/1
  PID Controller4/1 -> Scope33/1, Sum14/1
  Sum14/1 -> Divide2/1
  [I_boost] -> Scope12/1
  Constant6/1 -> Sum15/2
  Current Measurement1/1 -> [I_boost]
  [I_PV] -> Sum13/2
  Constant7/1 -> Goto26/1
  Constant8/1 -> Goto27/1
  Constant9/1 -> Goto28/1
  Constant10/1 -> [Iqref]
  Divide/1 -> Display/1, [mq]
  Divide1/1 -> Display1/1, [md]
  PID Controller/1 -> Sum1/2
  [ILOAD_q] -> Divide3/2
  Divide4/1 -> Sum9/2
  [ILOAD_d] -> Divide4/2
  [VLOAD_q] -> Divide4/1
  [ILOAD_d] -> Divide6/2
  Divide6/1 -> Sum6/1
  [ILOAD_q] -> Divide5/2
  [VLOAD_q] -> Divide5/1
  Constant/1 -> Goto5/1
  [Vdc] -> Divide2/2
  MATLAB Function1/1(iref) -> Goto24/1, Scope23/1, Display7/1
  From36/1 -> MATLAB Function1/2(Ipv)
  From37/1 -> MATLAB Function1/1(Vpv)
  Constant11/1 -> PV Array3/1
  PV Array2/1 -> [PV1]
  Voltage Measurement1/1 -> Scope24/1, Display10/1, [Vpv], To Workspace3/1
  Constant12/1 -> PV Array1/1
  Current Measurement/1 -> Display11/1, To Workspace/1, [I_PV]
  PV Array1/1 -> [PV2]
  Constant14/1 -> PV Array2/1
  Constant13/1 -> PV Array3/2, PV Array2/2, PV Array1/2
  PV Array3/1 -> [PV3]
  Bus Selector5/1 -> Product5/1, To Workspace4/1, Display22/1  "<I_PV>"
  From38/1 -> Bus Selector3/1
  Bus Selector4/1 -> Product4/1, To Workspace5/1, Display23/1  "<I_PV>"
  Bus Selector3/1 -> Product3/1, To Workspace6/1, Display24/1  "<I_PV>"
  Product3/1 -> Display25/1, To Workspace12/1
  Bus Selector3/2 -> To Workspace9/1, Product3/2, Display20/1  "<V_PV>"
  From42/1 -> Bus Selector4/1
  Product4/1 -> Display21/1, To Workspace11/1
  Bus Selector5/2 -> Display18/1, Product5/2, To Workspace7/1  "<V_PV>"
  Bus Selector4/2 -> Product4/2, To Workspace8/1, Display19/1  "<V_PV>"
  From43/1 -> Bus Selector5/1
  Product5/1 -> Display26/1, To Workspace10/1
  Bus Selector/2 -> Product1/2  "<I_PV>"
  [Vpv] -> Dot Product/1
  [PV3] -> Bus Selector/1
  Product2/1 -> Display29/1, Scope29/1
  Product1/1 -> Display28/1, Scope28/1
  [PV2] -> Bus Selector1/1
  Dot Product/1 -> To Workspace2/1, Scope26/1, Display27/1
  Bus Selector1/1 -> Scope27/2, Product2/1  "<V_PV>"
  [I_PV] -> Dot Product/2
  [PV1] -> Bus Selector2/1
  Bus Selector2/1 -> Scope27/3, Product6/1  "<V_PV>"
  Product6/1 -> Display17/1, Scope25/1
  Bus Selector1/2 -> Product2/2  "<I_PV>"
  Bus Selector2/2 -> Product6/2  "<I_PV>"
  Bus Selector/1 -> Scope27/1, Product1/1  "<V_PV>"
  [PV2] -> Display31/1
  [PV3] -> Display30/1
  [PV1] -> Display32/1
  [Vpv] -> Ppv/1
  Ptotal/1 -> To Workspace1/1, [Ppv_Losses], Display33/1, Scope30/1
  Plosses/1 -> Ptotal/2, Display35/1, Scope32/1
  Ppv/1 -> [Ppv], Ptotal/1
  Ipv^2/1 -> Plosses/1
  [I_PV] -> Ipv^2/2, Ipv^2/1, Ppv/2
  MATLAB Function4/1(I_pso) -> Display34/1, Goto32/1, Scope31/1
  Constant16/1 -> MATLAB Function4/5(Isc)
  Memory3/1 -> MATLAB Function4/2(Ipv)
  Constant17/1 -> MATLAB Function4/4(n)
  Memory2/1 -> MATLAB Function4/1(Vpv)
  From44/1 -> Memory3/1
  From67/1 -> Memory2/1
  Sum8/1 -> Plosses/2
  Sum10/1 -> Sum8/2
  (1-d)Rdi,on/1 -> Sum8/1
  Rdi,on/1 -> (1-d)Rdi,on/1
  (1-d)/1 -> (1-d)Rdi,on/2
  Constant18/1 -> (1-d)/1
  [mpv] -> (1-d)/2
  Rtr,on/1 -> Sum10/1
  Req/1 -> Sum10/2
  Memory1/1 -> MATLAB Function4/3(Ppv)
  From70/1 -> Memory1/1
  [Vpv] -> Sum14/2
  connections:
  Three-Phase Series RLC Branch/RConn1 -- Three-Phase V-I Measurement/RConn1
  Three-Phase V-I Measurement/LConn3 -- Two-Level Converter/LConn3
  Three-Phase Series RLC Branch/RConn3 -- Three-Phase V-I Measurement/RConn3
  Three-Phase V-I Measurement1/LConn3 -- Three-Phase Series RLC Branch/LConn3
  Three-Phase Series RLC Branch/RConn2 -- Three-Phase V-I Measurement/RConn2
  Ground/LConn1 -- Three-Phase Programmable Voltage Source/LConn1
  Three-Phase V-I Measurement1/LConn2 -- Three-Phase Series RLC Branch/LConn2
  Three-Phase V-I Measurement1/LConn1 -- Three-Phase Series RLC Branch/LConn1
  Three-Phase V-I Measurement/LConn2 -- Two-Level Converter/LConn2
  Three-Phase Programmable Voltage Source/RConn1 -- Three-Phase V-I Measurement1/RConn1
  Three-Phase V-I Measurement1/RConn3 -- Three-Phase Programmable Voltage Source/RConn3
  Three-Phase V-I Measurement1/RConn2 -- Three-Phase Programmable Voltage Source/RConn2
  Three-Phase V-I Measurement/LConn1 -- Two-Level Converter/LConn1
  Current Measurement1/RConn1 -- Series RLC Branch3/LConn1 -- Two-Level Converter/RConn1 -- Voltage Measurement2/LConn1
  Diode2/LConn1 -- PV Array2/RConn2 -- Voltage Measurement1/LConn2 -- RL2/RConn1 -- RL3/RConn1 -- IGBT/Diode1/RConn1 -- Series RLC Branch2/RConn1 -- Series RLC Branch3/RConn1 -- Voltage Measurement2/LConn2 -- Two-Level Converter/RConn2
  Diode1/RConn1 -- Series RLC Branch2/LConn1 -- Current Measurement1/LConn1
  Diode1/LConn1 -- IGBT/Diode1/LConn1 -- RL1/RConn1
  Current Measurement/LConn1 -- Diode4/RConn1 -- PV Array3/RConn1 -- Voltage Measurement1/LConn1 -- RL2/LConn1 -- RL3/LConn1
  PV Array1/RConn2 -- PV Array2/RConn1 -- Diode2/RConn1 -- Diode3/LConn1
  Diode4/LConn1 -- Diode3/RConn1 -- PV Array1/RConn1 -- PV Array3/RConn2
  Current Measurement/RConn1 -- RL1/LConn1

== matlab function pv_partial_shading_control/MATLAB Function1 ==
  settings: updateMethod=DISCRETE
  data: Vpv input; Ipv input; iref output
function iref = P_and_O(Vpv, Ipv)
    persistent Vold Pold iref_old Ipv_old;
    if isempty(Vold) % Initialize Vold, Pold, and iref_old with isempty
        Vold = 0;
        Pold = 0;
        iref_old =0;
        Ipv_old=0;
    end
    P = Vpv * Ipv;
    dP = P - Pold;
    dVpv = Vpv - Vold;
    dI = Ipv - Ipv_old;
    d = 0.01;
    if dP ~= 0
        if dP > 0
            if dI > 0
                iref = iref_old + d; % Change iref directly inside the if loop
            else
                iref = iref_old - d;
            end
        else
            if dI > 0
                iref = iref_old - d; % Change iref directly inside the if loop
            else
                iref = iref_old + d;
            end
        end
    else
        iref = iref_old;
    end
    Vold = Vpv;
    Pold = P;
    iref_old = iref;
    Ipv_old=Ipv;
end

== matlab function pv_partial_shading_control/MATLAB Function4 ==
  settings: updateMethod=DISCRETE
  data: Vpv input; I_pso output; Ipv input; Ppv input; n input; Isc input
function I_pso = PSO(Vpv,Ipv,Ppv,n,Isc) 

persistent u;          % current particle
persistent Icurrent;   % current I
persistent p;          % power
persistent pbest;
persistent I;          % current
persistent v;          % velocity (delta I)
persistent counter;
persistent gbest;


if isempty(counter)
    counter = 0;
end

if isempty(Icurrent)
    Icurrent = 0.7*Isc;
end

if isempty(gbest)
    gbest = Icurrent;
end

if isempty(p)
    p = zeros(n,1);
    for j = 1:n
         p(j) = -100000000;
    end
end

if isempty(v)
    v = zeros(n,1);
end

if isempty(pbest)
    pbest = zeros(n,1);
end

if isempty(u)
    u = 0;
end
if isempty(I)
    I = zeros(n, 1);
    for j = 1:n
         I(j) = 10 + rand() * (Isc - 10);  % Generate a random value between 20 and Isc
    end
end

if (counter >= 1 && counter < 500)
    I_pso = Icurrent;
    counter = counter + 1;
    return;
end

Vpv
Ipv
u

counter = 0;

if (u >= 1 && u <= n)
    p(u)
    if ((Ppv) > p(u))
        p(u) = Ppv;
        pbest(u) = Icurrent
    end
end

u = u + 1;

if u == (n+2)
    u = 1;
end

if (u >= 1 && u <= n)
    I_pso = I(u);
    Icurrent = I_pso;
    counter = 1;
    return;
elseif u == (n+1)
    [m,i] = max(p);
    pbest
    gbest = pbest(i)
    I_pso = gbest;
    Icurrent = I_pso;
    counter = 1;
    for j = 1:n
        v(j) = updatevelocity(v(j), pbest(j), I(j), gbest);
        I(j) = updateI(I(j), v(j));
    end
    v
    I
    return
else
    I_pso = 0.1*Isc;
end

end



function vfinal = updatevelocity(vel, pobest, I, gwbest)

w = 0.1;
c1 = 0.9;
c2 = 1.2;

vfinal = w*vel + c1*(pobest-I) + c2*(gwbest-I);

end


function Ifinal = updateI(I, vel)

Ifinal = I + vel;

end
